simulink model "EMplanner_cs2018a"  (R2018a)
settings: Solver=ode5  StartTime=0.0  StopTime=50  FixedStep=1/1000  RelTol=1e-3
PreLoadFcn:
  | mbxruntime.callbacks.PreLoadFcn(bdroot);
PostLoadFcn:
  | mbxruntime.callbacks.PostLoadFcn(bdroot);
InitFcn:
  | mbxruntime.callbacks.InitFcn(bdroot);
StartFcn:
  | mbxruntime.callbacks.StartFcn(bdroot);
StopFcn:
  | mbxruntime.callbacks.StopFcn(bdroot);
model workspace (MAT data in the model file):
  mbox_table : struct (value not decoded)
  model_closed = 0
  sim_status = 0
values from neighbouring files (symbols this model uses):
  c_factor = 43.75    [emplanner_init.m]
  cf = -175016    [emplanner_init.m]
  cr = -130634    [emplanner_init.m]
  global_path_x = [-2.9245 -1.92511774493 -0.926994634419 0.0698522493473 1.06541712279 2.05969835808 3.05269585569 4.04441007764 5.03484169183 6.02399144113 7.01186009523 7.99844843293 ... (1201 elements, 1201x1)]    [global_path.mat]
  global_path_y = [13.2143 13.2143 13.2143 13.2143 13.2143 13.2143 13.2143 13.2143 13.2143 13.2143 13.2143 13.2143 ... (1201 elements, 1201x1)]    [global_path.mat]
  KD_PID_distance = 0.0    (= 0)    [emplanner_init.m]
  KD_PID_speed = 0    [emplanner_init.m]
  KI_PID_distance = 0.0    (= 0)    [emplanner_init.m]
  KI_PID_speed = 0    [emplanner_init.m]
  KP_PID_distance = 0.5    [emplanner_init.m]
  KP_PID_speed = 1.8    [emplanner_init.m]
  la = 1.265    [emplanner_init.m]
  lb = 2.947-1.265    (= 1.682)    [emplanner_init.m]
  LQR_K1 = k(:,1)'    [emplanner_init.m]
  LQR_K2 = k(:,2)'    [emplanner_init.m]
  LQR_K3 = k(:,3)'    [emplanner_init.m]
  LQR_K4 = k(:,4)'    [emplanner_init.m]
  m = 2020    [emplanner_init.m]
  rack_displacement = [-39.14 , -37.2 , -35.29 , -33.43 , -31.6 , -29.81 , -28.06 , -26.34 , -24.66 ,      -23.01 , -21.38 , -19.79 , -18.23 , -16.69 , -15.18 , -13.7 , -12.23 , -10.8 , -9.38 , -7.98 ,     -6.61 , -5.25 , -3.91 , -2.59 , -1.29 , 0 , 1.27 , 2.54 , 3.78 , 5.02 , 6.24 , 7.46 , 8.66 ,      9.86 , 11.05 , 12.24 , 13.41 , 14.59 , 15.76 , 16.92 , 18.09 , 19.25 , 20.42 , 21.59 , 22.76 ,      23.93 , 25.11 , 26 ...(+26 chars)    [emplanner_init.m]
  right_wheel_ground = [-70 ,-67.2 , -64.4 , -61.6 , -58.8 , -56 , -53.2 , -50.4 , -47.6 , -44.8 , -42 ,      -39.2 , -36.4 , -33.6 , -30.8 , -28 , -25.2 , -22.4 , -19.6 , -16.8 , -14 , -11.2 , -8.4 , -5.6 ,      -2.8 , 0 , 2.8 , 5.6 , 8.4 , 11.2 , 14 , 16.8 , 19.6 , 22.4 , 25.2 , 28 , 30.8 , 33.6 , 36.4 ,      39.2 , 42 , 44.8 , 47.6 , 50.4 , 53.2 , 56 , 58.8 , 61.6 , 64.4 , 67.2 , 70 ]    [emplanner_init.m]
  vx_break_point = zeros(1,5000)    [emplanner_init.m]
undefined symbols (not defined in the file or in its folder): aubr, DiscIntNeverNeededParam, tablebr, vubr, warningInitialVelocity, x0
libraries: simulink x19, simulink_extras x5, PreScanSimulinkLibrary x4, Solver_SF x1
(part 3 of 5)

== system EMplanner_cs2018a/Audi_A8_Sedan_1/control module/control main/chassic steering system ==
  LQR_final_angle : Inport
  Constant : Constant  Value=la
  Constant1 : Constant  Value=lb
  Constant17 : Constant  Value=c_factor
  Divide : Product  Inputs=*/
  Gain3 : Gain  Gain=180/pi
  Gain4 : Gain  Gain=360
  MATLAB Function : MATLAB Function  TreatAsAtomicUnit=on
  Saturation : Saturate  UpperLimit=70  LowerLimit=-70
  Saturation1 : Saturate  UpperLimit=1.2217  LowerLimit=-1.2217
  transfer right wheel angle to rack displancement : Lookup_n-D  NumberOfTableDimensions=1  BreakpointsForDimension1=right_wheel_ground  Table=rack_displacement  InternalRulePriority=Speed  RndMeth=Simplest  InputSameDT=on
  lat_steer_sw[deg] : Outport
  wires:
  transfer right wheel angle to rack displancement/1 -> Divide/1
  Constant17/1 -> Divide/2
  Gain4/1 -> lat_steer_sw[deg]/1
  Divide/1 -> Gain4/1
  Saturation/1 -> transfer right wheel angle to rack displancement/1
  Constant/1 -> MATLAB Function/2(la)
  Gain3/1 -> Saturation/1
  Constant1/1 -> MATLAB Function/3(lb)
  LQR_final_angle/1 -> Saturation1/1
  Saturation1/1 -> MATLAB Function/1(u)
  MATLAB Function/1(right_steer) -> Gain3/1

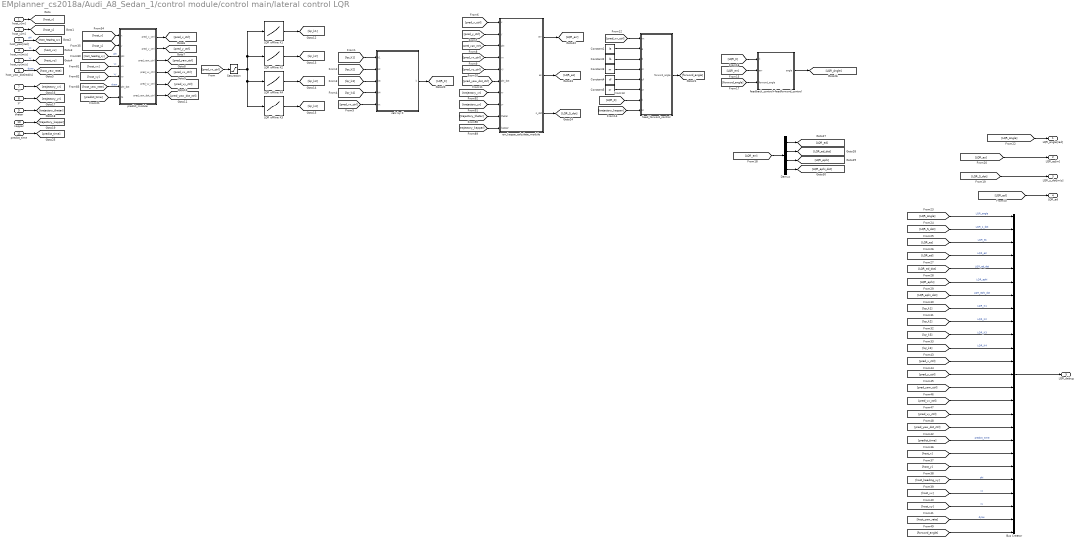
== system EMplanner_cs2018a/Audi_A8_Sedan_1/control module/control main/lateral control LQR ==
  host_x[m] : Inport
  host_y[m] : Inport  Port=2
  host_yaw[rad] : Inport  Port=3
  host_vx[m/s] : Inport  Port=4
  host_vy[m/s] : Inport  Port=5
  host_yaw_dot[rad/s] : Inport  Port=6
  xr : Inport  Port=7
  yr : Inport  Port=8
  thetar : Inport  Port=9
  kappar : Inport  Port=10
  predict_time : Inport  Port=11
  Bus Creator : BusCreator  Inputs=25
  Constant1 : Constant  Value=la
  Constant2 : Constant  Value=lb
  Constant3 : Constant  Value=m
  Constant4 : Constant  Value=cf
  Constant5 : Constant  Value=cr
  Demux : Demux
  LQR offline K1 : Lookup_n-D  NumberOfTableDimensions=1  BreakpointsForDimension1=vx_break_point  Table=LQR_K1  InternalRulePriority=Speed  RndMeth=Simplest  InputSameDT=on
  LQR offline K2 : Lookup_n-D  NumberOfTableDimensions=1  BreakpointsForDimension1=vx_break_point  Table=LQR_K2  InternalRulePriority=Speed  RndMeth=Simplest  InputSameDT=on
  LQR offline K3 : Lookup_n-D  NumberOfTableDimensions=1  BreakpointsForDimension1=vx_break_point  Table=LQR_K3  InternalRulePriority=Speed  RndMeth=Simplest  InputSameDT=on
  LQR offline K4 : Lookup_n-D  NumberOfTableDimensions=1  BreakpointsForDimension1=vx_break_point  Table=LQR_K4  InternalRulePriority=Speed  RndMeth=Simplest  InputSameDT=on
  Saturation : Saturate  UpperLimit=50  LowerLimit=0
  calc lqr K : MATLAB Function  TreatAsAtomicUnit=on
  err_kappa_calculate_module : MATLAB Function  TreatAsAtomicUnit=on
  feed_forword_control : MATLAB Function  TreatAsAtomicUnit=on
  feedback_control+feedforword_control : MATLAB Function  TreatAsAtomicUnit=on
  predict_module : MATLAB Function  TreatAsAtomicUnit=on
  LQR_angle[rad] : Outport  VectorParamsAs1DForOutWhenUnconnected=off
  LQR_es[m] : Outport  Port=2  VectorParamsAs1DForOutWhenUnconnected=off
  LQR_s_dot[m/s] : Outport  Port=3  VectorParamsAs1DForOutWhenUnconnected=off
  LQR_ed : Outport  Port=4  VectorParamsAs1DForOutWhenUnconnected=off
  LQR_debug : Outport  Port=5  VectorParamsAs1DForOutWhenUnconnected=off
  wires:
  [host_vy] -> predict_module/5(vy)  "vy"
  [host_x] -> predict_module/1(x)
  [host_yaw_rate] -> predict_module/6(phi_dot)  "dyaw"
  [host_vx] -> predict_module/4(vx)  "vx"
  [host_y] -> predict_module/2(y)
  [host_heading_xy] -> predict_module/3(phi)  "phi"
  [predict_time] -> predict_module/7(ts)
  host_x[m]/1 -> [host_x]
  host_y[m]/1 -> [host_y]
  host_yaw[rad]/1 -> [host_heading_xy]  "phi"
  host_vx[m/s]/1 -> [host_vx]  "vx"
  host_vy[m/s]/1 -> [host_vy]  "vy"
  host_yaw_dot[rad/s]/1 -> [host_yaw_rate]  "dyaw"
  predict_module/1(pred_x_ctrl) -> [pred_x_ctrl]
  predict_module/2(pred_y_ctrl) -> [pred_y_ctrl]
  predict_module/3(pred_yaw_ctrl) -> [pred_yaw_ctrl]
  predict_module/4(pred_vx_ctrl) -> [pred_vx_ctrl]
  predict_module/5(pred_vy_ctrl) -> [pred_vy_ctrl]
  predict_module/6(pred_yaw_dot_ctrl) -> [pred_yaw_dot_ctrl]
  [pred_vx_ctrl] -> Saturation/1
  LQR offline K1/1 -> [lqr_k1]
  LQR offline K2/1 -> [lqr_k2]
  LQR offline K4/1 -> [lqr_k3]
  LQR offline K3/1 -> [lqr_k4]
  [pred_vx_ctrl] -> calc lqr K/5(vx)
  [lqr_k4] -> calc lqr K/4(k4)
  [lqr_k3] -> calc lqr K/3(k3)
  [lqr_k2] -> calc lqr K/2(k2)
  [lqr_k1] -> calc lqr K/1(k1)
  [pred_x_ctrl] -> err_kappa_calculate_module/1(x)
  [pred_y_ctrl] -> err_kappa_calculate_module/2(y)
  [pred_yaw_ctrl] -> err_kappa_calculate_module/3(phi)
  [pred_vx_ctrl] -> err_kappa_calculate_module/4(vx)
  [pred_vy_ctrl] -> err_kappa_calculate_module/5(vy)
  [pred_yaw_dot_ctrl] -> err_kappa_calculate_module/6(phi_dot)
  xr/1 -> [trajectory_xr]
  yr/1 -> [trajectory_yr]
  thetar/1 -> [trajectory_thetar]
  kappar/1 -> [trajectory_kappar]
  [trajectory_xr] -> err_kappa_calculate_module/7(xr)
  [trajectory_yr] -> err_kappa_calculate_module/8(yr)
  [trajectory_kappar] -> err_kappa_calculate_module/10(kappar)
  [trajectory_thetar] -> err_kappa_calculate_module/9(thetar)
  [pred_vx_ctrl] -> feed_forword_control/1(vx)
  Constant1/1 -> feed_forword_control/2(a)
  Constant2/1 -> feed_forword_control/3(b)
  Constant3/1 -> feed_forword_control/4(m)
  Constant4/1 -> feed_forword_control/5(cf)
  Constant5/1 -> feed_forword_control/6(cr)
  calc lqr K/1(k) -> [LQR_K]
  [LQR_K] -> feed_forword_control/7(k)
  [trajectory_kappar] -> feed_forword_control/8(kr)
  feed_forword_control/1(forword_angle) -> [forword_angle]
  err_kappa_calculate_module/1(err) -> [LQR_err]
  [LQR_err] -> feedback_control+feedforword_control/2(err)
  [LQR_K] -> feedback_control+feedforword_control/1(k)
  [forword_angle] -> feedback_control+feedforword_control/3(forword_angle)
  [LQR_err] -> Demux/1
  err_kappa_calculate_module/2(es) -> [LQR_es]
  err_kappa_calculate_module/3(s_dot) -> [LQR_S_dot]
  [LQR_S_dot] -> LQR_s_dot[m/s]/1
  [LQR_es] -> LQR_es[m]/1
  Saturation/1 -> LQR offline K3/1, LQR offline K4/1, LQR offline K2/1, LQR offline K1/1
  predict_time/1 -> [predict_time]
  Bus Creator/1 -> LQR_debug/1
  feedback_control+feedforword_control/1(angle) -> [LQR_Angle]
  [LQR_Angle] -> LQR_angle[rad]/1
  [LQR_Angle] -> Bus Creator/1  "LQR_angle"
  [LQR_S_dot] -> Bus Creator/2  "LQR_s_dot"
  [LQR_es] -> Bus Creator/3  "LQR_es"
  Demux/1 -> [LQR_ed]
  Demux/2 -> [LQR_ed_dot]
  Demux/3 -> [LQR_ephi]
  Demux/4 -> [LQR_ephi_dot]
  [LQR_ed] -> Bus Creator/4  "LQR_ed"
  [LQR_ed_dot] -> Bus Creator/5  "LQR_ed_dot"
  [LQR_ephi] -> Bus Creator/6  "LQR_ephi"
  [LQR_ephi_dot] -> Bus Creator/7  "LQR_ephi_dot"
  [lqr_k1] -> Bus Creator/8  "LQR_K1"
  [lqr_k2] -> Bus Creator/9  "LQR_K2"
  [lqr_k3] -> Bus Creator/10  "LQR_K3"
  [lqr_k4] -> Bus Creator/11  "LQR_K4"
  [pred_x_ctrl] -> Bus Creator/12
  [pred_y_ctrl] -> Bus Creator/13
  [pred_yaw_ctrl] -> Bus Creator/14
  [pred_vx_ctrl] -> Bus Creator/15
  [pred_vy_ctrl] -> Bus Creator/16
  [pred_yaw_dot_ctrl] -> Bus Creator/17
  [predict_time] -> Bus Creator/18  "predict_time"
  [host_x] -> Bus Creator/19
  [host_y] -> Bus Creator/20
  [host_heading_xy] -> Bus Creator/21  "phi"
  [host_vx] -> Bus Creator/22  "vx"
  [host_vy] -> Bus Creator/23  "vy"
  [host_yaw_rate] -> Bus Creator/24  "dyaw"
  [forword_angle] -> Bus Creator/25
  [LQR_ed] -> LQR_ed/1

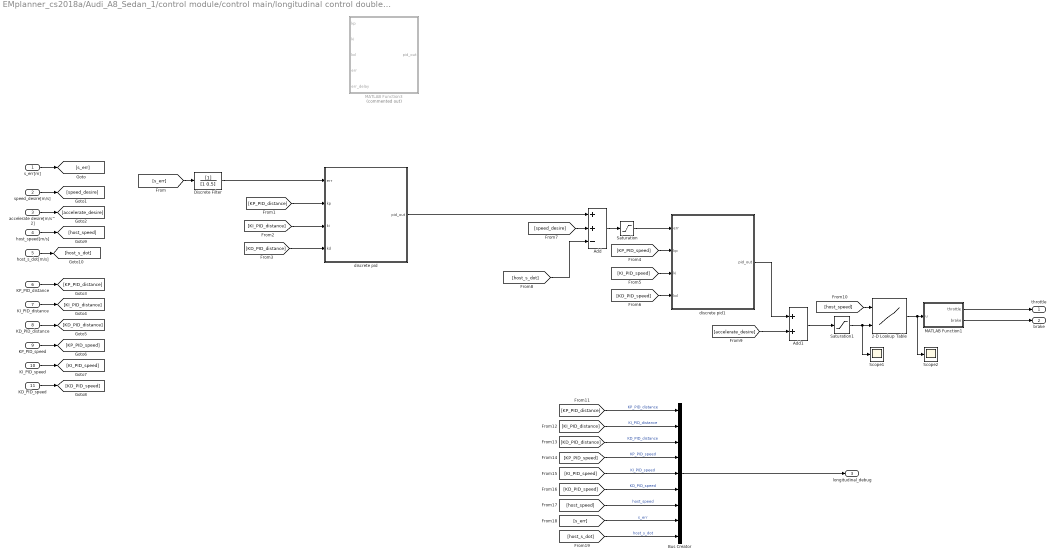
== system EMplanner_cs2018a/Audi_A8_Sedan_1/control module/control main/longitudinal control double PID ==
  s_err[m] : Inport
  speed_desire[m/s] : Inport  Port=2
  accelerate desire[m/s^2] : Inport  Port=3
  host_speed[m/s] : Inport  Port=4
  host_s_dot[m/s] : Inport  Port=5
  KP_PID_distance : Inport  Port=6
  KI_PID_distance : Inport  Port=7
  KD_PID_distance : Inport  Port=8
  KP_PID_speed : Inport  Port=9
  KI_PID_speed : Inport  Port=10
  KD_PID_speed : Inport  Port=11
  2-D Lookup Table : Lookup_n-D  BreakpointsForDimension1=vubr  BreakpointsForDimension2=aubr  Table=tablebr  InternalRulePriority=Speed  RndMeth=Simplest  InputSameDT=on
  Add : Sum  Inputs=++-
  Add1 : Sum
  Bus Creator : BusCreator  Inputs=9
  Discrete Filter : DiscreteFilter
  MATLAB Function1 : MATLAB Function  TreatAsAtomicUnit=on
  MATLAB Function3 : MATLAB Function  Commented=on  TreatAsAtomicUnit=on
  Saturation : Saturate  UpperLimit=45  LowerLimit=-45
  Saturation1 : Saturate  UpperLimit=5  LowerLimit=-8
  Scope1 : Scope
  Scope2 : Scope
  discrete pid : Subsystem
  discrete pid1 : Subsystem
  throttle : Outport
  brake : Outport  Port=2
  longitudinal_debug : Outport  Port=3
  wires:
  2-D Lookup Table/1 -> Scope2/1, MATLAB Function1/1(u)
  s_err[m]/1 -> [s_err]
  speed_desire[m/s]/1 -> [speed_desire]
  accelerate desire[m/s^2]/1 -> [accelerate_desire]
  KP_PID_distance/1 -> [KP_PID_distance]
  KI_PID_distance/1 -> [KI_PID_distance]
  KD_PID_distance/1 -> [KD_PID_distance]
  KP_PID_speed/1 -> [KP_PID_speed]
  KI_PID_speed/1 -> [KI_PID_speed]
  KD_PID_speed/1 -> [KD_PID_speed]
  [s_err] -> Discrete Filter/1
  host_speed[m/s]/1 -> [host_speed]
  [speed_desire] -> Add/2
  Add/1 -> Saturation/1
  Saturation/1 -> discrete pid1/1(err)
  discrete pid1/1(pid_out) -> Add1/1
  [accelerate_desire] -> Add1/2
  Add1/1 -> Saturation1/1
  Saturation1/1 -> Scope1/1, 2-D Lookup Table/2
  host_s_dot[m/s]/1 -> [host_s_dot]
  [host_s_dot] -> Add/3
  [host_speed] -> 2-D Lookup Table/1
  MATLAB Function1/1(throttle) -> throttle/1
  MATLAB Function1/2(brake) -> brake/1
  [KP_PID_distance] -> Bus Creator/1  "KP_PID_distance"
  [KI_PID_distance] -> Bus Creator/2  "KI_PID_distance"
  [KD_PID_distance] -> Bus Creator/3  "KD_PID_distance"
  [KP_PID_speed] -> Bus Creator/4  "KP_PID_speed"
  [KI_PID_speed] -> Bus Creator/5  "KI_PID_speed"
  [KD_PID_speed] -> Bus Creator/6  "KD_PID_speed"
  [host_speed] -> Bus Creator/7  "host_speed"
  [s_err] -> Bus Creator/8  "s_err"
  [host_s_dot] -> Bus Creator/9  "host_s_dot"
  Bus Creator/1 -> longitudinal_debug/1
  discrete pid/1(pid_out) -> Add/1
  Discrete Filter/1 -> discrete pid/1(err)
  [KP_PID_distance] -> discrete pid/2(kp)
  [KI_PID_distance] -> discrete pid/3(ki)
  [KD_PID_distance] -> discrete pid/4(kd)
  [KP_PID_speed] -> discrete pid1/2(kp)
  [KI_PID_speed] -> discrete pid1/3(ki)
  [KD_PID_speed] -> discrete pid1/4(kd)

== system EMplanner_cs2018a/Audi_A8_Sedan_1/control module/control main/understeer compensate ==
  LQR_angle : Inport
  lateral err : Inport  Port=2
  Add : Sum  Inputs=+-
  Gain : Gain  Gain=0.01
  Manual Switch : ManualSwitch
  LQR_final_angle : Outport
  wires:
  lateral err/1 -> Gain/1
  Add/1 -> Manual Switch/2
  Manual Switch/1 -> LQR_final_angle/1
  LQR_angle/1 -> Add/1, Manual Switch/1
  Gain/1 -> Add/2

== system EMplanner_cs2018a/Audi_A8_Sedan_2/Dynamics_Simple/Chassis/Bicycle_model_[XYZ] ==
  DeltaWheel_[rad] : Inport
  zFront_[m]_dzFront_[ms-1] : Inport  Port=2  PortDimensions=2
  zRear_[m]_dzRear_[ms-1] : Inport  Port=3  PortDimensions=2
  BrakePressure_[bar] : Inport  Port=4
  DriveTorque_[Nm] : Inport  Port=5
  v0_[ms-1] : Inport  Port=6
  |vx|_[ms-1] : Inport  Port=7
  Fy_rear_[N] : Inport  Port=8
  Fy_front_[N] : Inport  Port=9
  Demux : Demux  Outputs=2
  Demux1 : Demux  Outputs=2
  Fyi --> Fy / Mz : Subsystem
  X_Motion : Subsystem
  Y & Yaw_Motion : Subsystem
  "Z, Pitch_Motion & Roll_Motion" : Subsystem
  |vx|_[ms-1]1 : Outport
  vy_[ms-1] : Outport  Port=2
  vz_[ms-1] : Outport  Port=3
  RollAngle_[rad] : Outport  Port=4
  RollRate_[rads-1] : Outport  Port=5
  YawAngle_[rads-1] : Outport  Port=6
  Vx_[ms-1] : Outport  Port=7
  PitchAngle_[rad] : Outport  Port=8
  YawAngle_[rad] : Outport  Port=9
  ax_[ms-2] : Outport  Port=10
  ay_[ms-2] : Outport  Port=11
  wires:
  Fyi --> Fy / Mz/1(Fy_[N]) -> Y & Yaw_Motion/2(Fy_[N])  "Fy_[N]"
  Fyi --> Fy / Mz/2(Mz_[Nm]) -> Y & Yaw_Motion/3(Mz_[Nm])  "Mz_[Nm]"
  Y & Yaw_Motion/1(|vx|_[ms-1]1) -> |vx|_[ms-1]1/1  "|vx|_[ms-1]"
  Y & Yaw_Motion/2(vy_[ms-1]) -> vy_[ms-1]/1  "vy_[ms-1]"
  Y & Yaw_Motion/5(YawAngle_[rad]) -> YawAngle_[rad]/1  "YawAngle_[rad]"
  v0_[ms-1]/1 -> X_Motion/3(v0_[ms-1])  "v0_[ms-1]"
  BrakePressure_[bar]/1 -> X_Motion/2(BrakePressure_[bar])  "BrakePressure_[bar]"
  DriveTorque_[Nm]/1 -> X_Motion/1(DriveTorque_[Nm])  "DriveTorque_[Nm]"
  X_Motion/2(ax_[ms-2]) -> ax_[ms-2]/1, [ax]  "ax_[ms-2]"
  X_Motion/1(vx_[ms-1]) -> Vx_[ms-1]/1, [vx]  "vx_[ms-1]"
  [ax] -> "Z, Pitch_Motion & Roll_Motion"/3(ax)
  Demux/1 -> "Z, Pitch_Motion & Roll_Motion"/5(zFront_[m])
  Demux/2 -> "Z, Pitch_Motion & Roll_Motion"/6(dzFront_[ms-1])
  Demux1/1 -> "Z, Pitch_Motion & Roll_Motion"/7(zRear_[m])
  Demux1/2 -> "Z, Pitch_Motion & Roll_Motion"/8(dzRear_[ms-1])
  zRear_[m]_dzRear_[ms-1]/1 -> Demux1/1
  zFront_[m]_dzFront_[ms-1]/1 -> Demux/1
  "Z, Pitch_Motion & Roll_Motion"/2(vz_[ms-1]) -> vz_[ms-1]/1  "vz_[ms-1]"
  DeltaWheel_[rad]/1 -> Fyi --> Fy / Mz/1(DeltaWheel_[rad])
  Fy_front_[N]/1 -> Fyi --> Fy / Mz/2(Fy_f_[N])
  Fy_rear_[N]/1 -> Fyi --> Fy / Mz/3(Fy_r_[N])
  |vx|_[ms-1]/1 -> Y & Yaw_Motion/1(|vx|_[ms-1])
  Y & Yaw_Motion/3(ay_[ms-2]) -> [ay], ay_[ms-2]/1  "ay_[ms-2]"
  [ay] -> "Z, Pitch_Motion & Roll_Motion"/4(ay)
  "Z, Pitch_Motion & Roll_Motion"/3(RollAngle_[rad]) -> RollAngle_[rad]/1  "RollAngle_[rad]"
  "Z, Pitch_Motion & Roll_Motion"/4(RollRate_[rads-1]) -> RollRate_[rads-1]/1  "RollRate_[rads-1]"
  [dYaw] -> "Z, Pitch_Motion & Roll_Motion"/2(dYaw)
  [vx] -> "Z, Pitch_Motion & Roll_Motion"/1(vx)
  Y & Yaw_Motion/4(dYawAngle_[rads-1]) -> YawAngle_[rads-1]/1, [dYaw]  "dYawAngle_[rads-1]"
  "Z, Pitch_Motion & Roll_Motion"/1(pitchAngle_[rad]) -> PitchAngle_[rad]/1  "PitchAngle_[rad]"

== system EMplanner_cs2018a/Audi_A8_Sedan_2/Dynamics_Simple/Chassis/FrontTyre ==
  note: alpha limiter
      | [-1 ... 1]
  note: relax_on
      | ON: 1
      | OFF: 0
  note: MOTORCYCLE ONLY
  note: VEHICLE + MOTORCYCLE
  DeltaWheel_[rad] : Inport
  |vx|_[ms-1] : Inport  Port=2
  vy_[ms-1] : Inport  Port=3
  dYawAngle_[rads-1] : Inport  Port=4
  RollAngle_[rad] : Inport  Port=5
  AlphaFront : Subsystem
  Compare To Zero : simulink/Logic and Bit Operations/Compare To Zero  relop===  OutDataTypeStr=boolean  ZeroCross=off
  Configurable Subsystem : Subsystem  BlockChoice=Integrator  mask{ComputationMode=ComputationMode}
      mask prompts: ComputationMode "Computation mode:"
      mask init:
      | SetComputationMode(gcb,ComputationMode);
      settings: AttributesFormatString=%<BlockChoice>  OpenFcn=BringToFront(gcb);  MemberBlocks=Discrete-Time Integrator,Integrator
      settings: TemplateBlock=|
      | PreScanSimulinkLibrary/Configurable Subsystems/integral with reset and limits
      | for slip angle/Configurable
      | Subsystem
  Configurable Subsystem1 : Subsystem  BlockChoice=Integrator  mask{ComputationMode=ComputationMode}
      mask prompts: ComputationMode "Computation mode:"
      mask init:
      | SetComputationMode(gcb,ComputationMode);
      settings: AttributesFormatString=%<BlockChoice>  OpenFcn=BringToFront(gcb);  MemberBlocks=Discrete-Time Integrator,Integrator
      settings: TemplateBlock=|
      | PreScanSimulinkLibrary/Configurable Subsystems/integral with reset/Configurable
      | Subsystem
  Constant : Constant  Value=p.relax_on
  Constant1 : Constant  Value=p.relax_on
  Constant2 : Constant  Value=p.VehMCSwitch
  Data Type Conversion : DataTypeConversion  OutDataTypeStr=double
  If MC : simulink/Logic and Bit Operations/Compare To Constant  relop===  const=2  OutDataTypeStr=uint8  ZeroCross=off
  K_gamma_front : Gain  Gain=p.Kgfront
  Linl : Fcn  Expr=(u(4) - u(5))/p.sigma_front*u(1)
  Linl1 : Fcn  Expr=(u(4) - u(5))/p.sigma_front*u(1)
  Mux1 : Mux  Inputs=3
  Mux2 : Mux  Inputs={3,1,1}
  Mux3 : Mux  Inputs={3,1,1}
  Prevent_instability_at_low_Vx : Subsystem
  Product : Product  RndMeth=Zero
  Sum : Sum  Inputs=|++  InputSameDT=on  SaturateOnIntegerOverflow=on  OutDataTypeStr=Inherit: Same as first input
  Sum1 : Sum  Inputs=|++
  Switch : Switch  Threshold=0.5  SaturateOnIntegerOverflow=on  InputSameDT=on
  Switch1 : Switch  Threshold=0.5  SaturateOnIntegerOverflow=on  InputSameDT=on
  alg.loop : Memory
  due to sign convention : Gain  Gain=-1  SaturateOnIntegerOverflow=on  OutDataTypeStr=Inherit: Same as input  ParamDataTypeStr=Inherit: Same as input
  front_tyre : Gain  Gain=p.Kfront
  FyFront_[N] : Outport
  wires:
  Prevent_instability_at_low_Vx/1(alpha [rad]) -> Mux2/2, Switch/3
  Sum/1 -> Prevent_instability_at_low_Vx/1(alpha[rad])  "AlphaStatFront_[rad]"
  Switch/1 -> front_tyre/1  "AlphaFront_[rad]"
  Constant/1 -> Switch/2
  Sum1/1 -> FyFront_[N]/1  "FyFront_[N]"
  Mux2/1 -> Linl/1
  Linl/1 -> Configurable Subsystem/1(In1)
  Configurable Subsystem/1(Out1) -> Mux2/3, Switch/1  "AlphaRelaxFront_[rad]"
  AlphaFront/1(Alpha) -> Sum/1
  Mux1/1 -> Prevent_instability_at_low_Vx/2(In), AlphaFront/1(In), Mux2/1, Mux3/1
  |vx|_[ms-1]/1 -> Mux1/1, Compare To Zero/1
  vy_[ms-1]/1 -> Mux1/2
  dYawAngle_[rads-1]/1 -> Mux1/3
  alg.loop/1 -> Switch1/3
  Configurable Subsystem1/1(Out1) -> Mux3/3, Switch1/1  "GammaRelaxFront_[rad]"
  Linl1/1 -> Configurable Subsystem1/1(In1)
  Mux3/1 -> Linl1/1
  Constant1/1 -> Switch1/2
  due to sign convention/1 -> alg.loop/1, Mux3/2  "GammaStatFront_[rad]"
  RollAngle_[rad]/1 -> due to sign convention/1
  front_tyre/1 -> Sum1/1
  Constant2/1 -> If MC/1
  If MC/1 -> Data Type Conversion/1
  K_gamma_front/1 -> Product/1
  Product/1 -> Sum1/2
  Data Type Conversion/1 -> Product/2
  Compare To Zero/1 -> [reset]
  [reset] -> Configurable Subsystem/2(In2)
  [reset] -> Configurable Subsystem1/2(In2)
  DeltaWheel_[rad]/1 -> Sum/2  "DeltaWheel_[rad]"
  Switch1/1 -> K_gamma_front/1  "GammaFront_[rad]"

== system EMplanner_cs2018a/Audi_A8_Sedan_2/Dynamics_Simple/Chassis/MuxDynState ==
  note: The position inputs are computed by the
      | integrated velocity.
  note: mode: Dynamics
      | VelVEHICLE
      | wrt VEH
  note: AnglesVEHICLE
      | wrtGLOB
  vx [ms-1] : Inport
  vy [ms-1] : Inport  Port=2
  vz [ms-1] : Inport  Port=3
  R [rad] : Inport  Port=4
  P [rad] : Inport  Port=5
  Y [rad] : Inport  Port=6
  Configurable Subsystem1 : Subsystem  BlockChoice=Integrator  mask{ComputationMode=ComputationMode}
      mask prompts: ComputationMode "Computation mode:"
      mask init:
      | SetComputationMode(gcb,ComputationMode);
      settings: AttributesFormatString=%<BlockChoice>  OpenFcn=BringToFront(gcb);  MemberBlocks=Discrete-Time Integrator,Integrator
      settings: TemplateBlock=|
      | PreScanSimulinkLibrary/Configurable Subsystems/integral/Configurable
      | Subsystem1
  Ground : Ground
  Ground1 : Ground
  Mux : Mux  Inputs=[3 3 3]
  Mux1 : Mux  Inputs=3
  Mux2 : Mux  Inputs=3
  Transformation_BODY2GLOBAL : Subsystem
  mux3 : Mux  Inputs=3
  State : Outport
  wires:
  Ground1/1 -> mux3/2  "pitch"
  Y [rad]/1 -> Mux2/3, mux3/3  "yaw"
  P [rad]/1 -> Mux2/2
  R [rad]/1 -> Mux2/1
  vz [ms-1]/1 -> Mux1/3
  vy [ms-1]/1 -> Mux1/2
  vx [ms-1]/1 -> Mux1/1
  Mux2/1 -> Mux/3
  Transformation_BODY2GLOBAL/1(Vvector_GLOBAL_[m/s]) -> Configurable Subsystem1/1(In1), Mux/2  "VelVEH wrt  GLOB"
  mux3/1 -> Transformation_BODY2GLOBAL/2(angles_BODYwrtGLOB_[rad])
  Ground/1 -> mux3/1  "roll"
  Mux/1 -> State/1
  Mux1/1 -> Transformation_BODY2GLOBAL/1(Vvector_BODY_[m/s])
  Configurable Subsystem1/1(Out1) -> Mux/1  "PosVEH wrt  GLOB"

== system EMplanner_cs2018a/Audi_A8_Sedan_2/Dynamics_Simple/Chassis/Power Assisted Steering ==
  note: MOTORCYCLE
  note: VEHICLE
  note: Reverse steering direction for negative velocities
  Vx_[ms-1] : Inport
  Delta_in_[deg] : Inport  Port=2
  Constant : Constant
  Constant1 : Constant  Value=p.VehMCSwitch
  Lookup Table : Lookup  InputValues=[0 35 45 100]  Table=[1 1 0.2 0.2]
  Multiport Switch : MultiPortSwitch  Inputs=2
  Product : Product  Inputs=3  RndMeth=Zero
  Sign : Signum
  Delta_out_[deg] : Outport
  wires:
  Vx_[ms-1]/1 -> Lookup Table/1, Sign/1
  Delta_in_[deg]/1 -> Product/3
  Constant1/1 -> Multiport Switch/1
  Constant/1 -> Multiport Switch/3
  Lookup Table/1 -> Multiport Switch/2
  Multiport Switch/1 -> Product/2
  Product/1 -> Delta_out_[deg]/1
  Sign/1 -> Product/1

== system EMplanner_cs2018a/Audi_A8_Sedan_2/Dynamics_Simple/Chassis/RearTyre ==
  note: alpha limiter
      | [-1 ... 1]
  note: relax_on
      | ON: 1
      | OFF: 0
  note: MOTORCYCLE ONLY
  note: VEHICLE + MOTORCYCLE
  |vx|_[ms-1] : Inport
  vy_[ms-1] : Inport  Port=2
  dpsi_[rads-1] : Inport  Port=3
  RollAngle_[rad] : Inport  Port=4
  AlphaRear : Subsystem
  Compare To Zero : simulink/Logic and Bit Operations/Compare To Zero  relop===  OutDataTypeStr=boolean  ZeroCross=off
  Configurable Subsystem : Subsystem  BlockChoice=Integrator  mask{ComputationMode=ComputationMode}
      mask prompts: ComputationMode "Computation mode:"
      mask init:
      | SetComputationMode(gcb,ComputationMode);
      settings: AttributesFormatString=%<BlockChoice>  OpenFcn=BringToFront(gcb);  MemberBlocks=Discrete-Time Integrator,Integrator
      settings: TemplateBlock=|
      | PreScanSimulinkLibrary/Configurable Subsystems/integral with reset/Configurable
      | Subsystem
  Configurable Subsystem1 : Subsystem  BlockChoice=Integrator  mask{ComputationMode=ComputationMode}
      mask prompts: ComputationMode "Computation mode:"
      mask init:
      | SetComputationMode(gcb,ComputationMode);
      settings: AttributesFormatString=%<BlockChoice>  OpenFcn=BringToFront(gcb);  MemberBlocks=Discrete-Time Integrator,Integrator
      settings: TemplateBlock=|
      | PreScanSimulinkLibrary/Configurable Subsystems/integral with reset and limits
      | for slip angle/Configurable
      | Subsystem
  Constant1 : Constant  Value=p.relax_on
  Constant2 : Constant  Value=p.relax_on
  Constant3 : Constant  Value=p.VehMCSwitch
  Data Type Conversion : DataTypeConversion  OutDataTypeStr=double
  If MC : simulink/Logic and Bit Operations/Compare To Constant  relop===  const=2  OutDataTypeStr=uint8  ZeroCross=off
  K_gamma_rear : Gain  Gain=p.Kgrear
  Linl : Fcn  Expr=(u(4) - u(5))/p.sigma_rear*u(1)
  Linl1 : Fcn  Expr=(u(4) - u(5))/p.sigma_rear*u(1)
  Mux1 : Mux  Inputs=3
  Mux2 : Mux  Inputs={3,1,1}
  Mux3 : Mux  Inputs={3,1,1}
  Prevent_instability_at_low_Vx : PreScanSimulinkLibrary/Simple_Vehicle_Dynamics/Chassis/FrontTyre/Prevent_instability_at_low_Vx  SystemSampleTime=-1  Latency=0  AutoFrameSizeCalculation=off
  Product : Product  RndMeth=Zero
  Sum1 : Sum  Inputs=|++
  Switch1 : Switch  Threshold=0.5  SaturateOnIntegerOverflow=on  InputSameDT=on
  Switch2 : Switch  Threshold=0.5  SaturateOnIntegerOverflow=on  InputSameDT=on
  alg.loop : Memory
  due to sign convention : Gain  Gain=-1  SaturateOnIntegerOverflow=on  OutDataTypeStr=Inherit: Same as input  ParamDataTypeStr=Inherit: Same as input
  rear_tyre : Gain  Gain=p.Krear
  FyRear_[N] : Outport
  wires:
  Prevent_instability_at_low_Vx/1 -> Switch1/3, Mux2/2
  AlphaRear/1(Alpha) -> Prevent_instability_at_low_Vx/1  "AlphaStatRear_[rad]"
  Switch1/1 -> rear_tyre/1  "AlphaRear_[rad]"
  Constant1/1 -> Switch1/2
  Sum1/1 -> FyRear_[N]/1  "FyRear_[N]"
  Mux2/1 -> Linl/1
  Linl/1 -> Configurable Subsystem1/1(In1)
  Configurable Subsystem1/1(Out1) -> Mux2/3, Switch1/1  "AlphaRelaxRear_[rad]"
  Mux1/1 -> Prevent_instability_at_low_Vx/2, AlphaRear/1(In), Mux2/1, Mux3/1
  |vx|_[ms-1]/1 -> Mux1/1, Compare To Zero/1
  vy_[ms-1]/1 -> Mux1/2
  dpsi_[rads-1]/1 -> Mux1/3
  alg.loop/1 -> Switch2/3
  Configurable Subsystem/1(Out1) -> Mux3/3, Switch2/1  "GammaRelaxRear_[rad]"
  Linl1/1 -> Configurable Subsystem/1(In1)
  Mux3/1 -> Linl1/1
  Constant2/1 -> Switch2/2
  due to sign convention/1 -> alg.loop/1, Mux3/2  "GammaStatRear_[rad]"
  RollAngle_[rad]/1 -> due to sign convention/1
  Constant3/1 -> If MC/1
  If MC/1 -> Data Type Conversion/1
  Product/1 -> Sum1/2
  Data Type Conversion/1 -> Product/2
  K_gamma_rear/1 -> Product/1
  rear_tyre/1 -> Sum1/1
  Compare To Zero/1 -> [reset]
  [reset] -> Configurable Subsystem1/2(In2)
  [reset] -> Configurable Subsystem/2(In2)
  Switch2/1 -> K_gamma_rear/1  "GammaFront_[rad]"

== system EMplanner_cs2018a/Audi_A8_Sedan_2/Dynamics_Simple/Engine/Configurable Subsystem ==
  In1 : Inport
  Rate Limiter : TransferFcn  Denominator=[0.1 1]
  Out1 : Outport
  wires:
  In1/1 -> Rate Limiter/1
  Rate Limiter/1 -> Out1/1

== system EMplanner_cs2018a/Audi_A8_Sedan_2/Dynamics_Simple/Engine/Configurable Subsystem1 ==
  In1 : Inport
  Integrator : Integrator  InitialCondition=p.rot_ini  LimitOutput=on  UpperSaturationLimit=p.rot_upp  LowerSaturationLimit=p.rot_low
  Out1 : Outport
  wires:
  In1/1 -> Integrator/1
  Integrator/1 -> Out1/1

== system EMplanner_cs2018a/Audi_A8_Sedan_2/Dynamics_Simple/Gear: Auto Manual/If Action Subsystem ==
  In1 : Inport
  Action Port : ActionPort  PropagateVarSize=During execution
  Out1 : Outport
  wires:
  In1/1 -> Out1/1

== system EMplanner_cs2018a/Audi_A8_Sedan_2/Dynamics_Simple/Gear: Auto Manual/If Action Subsystem1 ==
  In1 : Inport
  Action Port : ActionPort  PropagateVarSize=During execution
  Out1 : Outport
  wires:
  In1/1 -> Out1/1

== system EMplanner_cs2018a/Audi_A8_Sedan_2/Dynamics_Simple/ShiftLogic/Detect Increase ==
  GearNr_[-] : Inport
  In2 : Inport  Port=2
  Constant : Constant
  Data Type Conversion : DataTypeConversion  OutDataTypeStr=double
  Data Type Conversion1 : DataTypeConversion  OutDataTypeStr=double
  Detect Increase : simulink/Logic and Bit Operations/Detect Increase  vinit=1  OutDataTypeStr=uint8
  If : If  NumInputs=2  IfExpression="u1==1 &  u2==1"
  If V0 higher of the from 2->3 shifting velocity : Subsystem  TreatAsAtomicUnit=on
  Merge : Merge
  Other : Subsystem  TreatAsAtomicUnit=on
  Out1 : Outport
  wires:
  If/2 -> Other/Action
  If V0 higher of the from 2->3 shifting velocity/1(Out1) -> Merge/1
  Other/1(Out1) -> Merge/2
  Detect Increase/1 -> Data Type Conversion/1
  Merge/1 -> Out1/1
  If/1 -> If V0 higher of the from 2->3 shifting velocity/Action
  Data Type Conversion1/1 -> If/2
  Data Type Conversion/1 -> If/1
  Constant/1 -> If V0 higher of the from 2->3 shifting velocity/1(In1)
  GearNr_[-]/1 -> Detect Increase/1
  In2/1 -> Data Type Conversion1/1, Other/1(In1)

== system EMplanner_cs2018a/Audi_A8_Sedan_2/Dynamics_Simple/ShiftLogic/If Action Neutral ==
  In1 : Inport
  Action Port : ActionPort  InitializeStates=reset  PropagateVarSize=During execution
  Out1 : Outport
  wires:
  In1/1 -> Out1/1

== system EMplanner_cs2018a/Audi_A8_Sedan_2/Dynamics_Simple/ShiftLogic/If Action Normal ==
  In1 : Inport
  Action Port : ActionPort  InitializeStates=reset  PropagateVarSize=During execution
  Out1 : Outport
  wires:
  In1/1 -> Out1/1

== system EMplanner_cs2018a/Audi_A8_Sedan_2/Dynamics_Simple/ShiftLogic/If Action Reverse ==
  In1 : Inport
  Action Port : ActionPort  InitializeStates=reset  PropagateVarSize=During execution
  Out1 : Outport
  wires:
  In1/1 -> Out1/1

== system EMplanner_cs2018a/Audi_A8_Sedan_2/Dynamics_Simple/Transmission/Torque_Converter ==
  note: <= 0
  note: > 0
  note: To compensate for no hydraulic connection when in neutral gear
  nEngine_[rpm] : Inport
  nTransmission_[rpm] : Inport  Port=2
  Gear nr : Inport  Port=3
  Compare To Constant : simulink/Logic and Bit Operations/Compare To Constant  relop=<=  const=1  OutDataTypeStr=uint8  ZeroCross=off
  Compare To Zero : simulink/Logic and Bit Operations/Compare To Zero  relop=~=  OutDataTypeStr=uint8  ZeroCross=off
  Constant : Constant  Value=1/50
  Constant1 : Constant
  Constant2 : Constant
  Drag : Gain  Gain=-1
  FactorK : Lookup  InputValues=p.speedratio  Table=p.Kfactor*p.Kcorr  SaturateOnIntegerOverflow=on
  Impeller : Fcn  Expr=u^2
  Product : Product  RndMeth=Zero
  Product1 : Product  RndMeth=Zero
  Quotient : Product  Inputs=*/  InputSameDT=on  SaturateOnIntegerOverflow=on  OutDataTypeStr=Inherit: Same as first input
  SpeedRatio : Product  Inputs=*/  InputSameDT=on  SaturateOnIntegerOverflow=on  OutDataTypeStr=Inherit: Same as first input
  Sum : Sum  Inputs=|+-
  Switch : Switch  Criteria=u2 ~= 0  Threshold=0.5
  Switch1 : Switch  Criteria=u2 ~= 0
  TorqueRatio : Lookup  InputValues=[p.speedratio 1]  Table=[p.Torqueratio 0]  SaturateOnIntegerOverflow=on
  Turbine : Product  InputSameDT=on  SaturateOnIntegerOverflow=on  OutDataTypeStr=Inherit: Same as first input
  rpm2rads-1 : Gain  Gain=2*pi/60
  ImpellerTorque_[Nm] : Outport  InitialOutput=0
  TurbineTorque_[Nm] : Outport  Port=2  InitialOutput=0
  wires:
  rpm2rads-1/1 -> Quotient/1
  Turbine/1 -> Switch1/1
  TorqueRatio/1 -> Turbine/2
  Compare To Constant/1 -> Switch1/2
  Constant2/1 -> Sum/2
  Sum/1 -> Drag/1
  Drag/1 -> Switch1/3
  Product1/1 -> TurbineTorque_[Nm]/1
  Switch1/1 -> Product1/2
  Compare To Zero/1 -> Switch/2
  Gear nr/1 -> Compare To Zero/1
  Constant1/1 -> Switch/1
  Constant/1 -> Switch/3
  Switch/1 -> Product1/1, Product/1
  Product/1 -> ImpellerTorque_[Nm]/1
  Quotient/1 -> Impeller/1
  FactorK/1 -> Quotient/2
  SpeedRatio/1 -> FactorK/1, Sum/1, Compare To Constant/1, TorqueRatio/1
  Impeller/1 -> Turbine/1, Product/2
  nEngine_[rpm]/1 -> SpeedRatio/2, rpm2rads-1/1
  nTransmission_[rpm]/1 -> SpeedRatio/1

== system EMplanner_cs2018a/Audi_A8_Sedan_2/Dynamics_Simple/Transmission/Transmission_Ratio ==
  tTransmissionIn_[Nm] : Inport
  GearNr_[-] : Inport  Port=2
  nTransmissionOut_[rpm] : Inport  Port=3
  Ensure positive TransmissionRPM : Abs
  If : If  IfExpression=u1 == 0  ElseIfExpressions=u1 == -1
  If Action Neutral : Subsystem  TreatAsAtomicUnit=on
  If Action Normal : Subsystem  TreatAsAtomicUnit=on
  If Action Reverse : Subsystem  TreatAsAtomicUnit=on
  Merge : Merge  Inputs=3
  OutputTorque = 0 : Constant  Value=0
  Product : Product  InputSameDT=on  SaturateOnIntegerOverflow=on  OutDataTypeStr=Inherit: Same as first input
  Product1 : Product  InputSameDT=on  SaturateOnIntegerOverflow=on  OutDataTypeStr=Inherit: Same as first input
  Transmission Gear ratios : Lookup  InputValues=p.tr_in  Table=p.tr_out  SaturateOnIntegerOverflow=on
  tTransmissionOut_[Nm] : Outport  InitialOutput=0
  nTransmissionIn_[rpm] : Outport  Port=2  InitialOutput=0
  wires:
  GearNr_[-]/1 -> Transmission Gear ratios/1, If/1
  If/3 -> If Action Normal/Action
  If/2 -> If Action Reverse/Action
  If Action Normal/1(Out1) -> Merge/3
  If Action Reverse/1(Out1) -> Merge/2
  If/1 -> If Action Neutral/Action
  If Action Neutral/1(Out1) -> Merge/1
  Product1/1 -> Ensure positive TransmissionRPM/1
  Merge/1 -> tTransmissionOut_[Nm]/1
  Product/1 -> If Action Reverse/1(In1), If Action Normal/1(In1)
  OutputTorque = 0/1 -> If Action Neutral/1(In1)
  Transmission Gear ratios/1 -> Product/2, Product1/1
  nTransmissionOut_[rpm]/1 -> Product1/2
  tTransmissionIn_[Nm]/1 -> Product/1
  Ensure positive TransmissionRPM/1 -> nTransmissionIn_[rpm]/1

== system EMplanner_cs2018a/Audi_A8_Sedan_2/PathFollower_Preview_1/LateralController/CTRL REFERENCES ==
  note: REFERENCE POSITION BASED POSITION CTRL
  Pos x,y,Y [m,m,rad] : Inport
  Position Preview Distance [m] : Inport  Port=2
  TrajOffset [m,m,rad] : Inport  Port=3
  ActorOffset_Left(+) / Right(-)_[m] : Inport  Port=4
  Calculate Lateral Error : Subsystem
      mask Display:
      | port_label('input',1,'pvp');
      | port_label('input',2,'TrajOffset_x_y_Y');
      | port_label('input',3,'ActorOffset_Left_Right');
      | port_label('input',4,'p0');
      | port_label('input',5,'PreviewDistance');
      | port_label('output',1,'dist_psvehicle');
  Calculate Preview Point (pvp) by extrapolating current Vehicle Position (p0) with Preview Distance and Vehicle Orientation : Subsystem
  Find Reference Point (pref0) on Trajectory closest to P0 Point (p0) : Subsystem
      mask Display:
      | port_label('input',1,'pvp');
      | port_label('input',2,'TrajOffset_x_y_Y');
      | port_label('input',3,'ActorOffset_Left_Right');
      | port_label('input',4,'p0');
      | port_label('output',1,'Actor_traj_distance');
      | port_label('output',2,'Actor_traj_angle');
  Mux1 : Mux  Inputs=2
  Selector2 : Selector  InputPortWidth=3  IndexOptions=Index vector (dialog)  Indices=[1 2]  OutputSizes=1
  Terminator : Terminator
  Actor/Traj_distance [m] : Outport
  Actor/Traj_angle [deg] : Outport  Port=2
  e_Lat [m] : Outport  Port=3
  wires:
  Mux1/1 -> Calculate Lateral Error/1(In1), Find Reference Point (pref0) on Trajectory closest to P0 Point (p0)/1(In1)
  Pos x,y,Y [m,m,rad]/1 -> Calculate Preview Point (pvp) by extrapolating current Vehicle Position (p0) with Preview Distance and Vehicle Orientation/2(x,y,Y Demux [m,m,rad]), Find Reference Point (pref0) on Trajectory closest to P0 Point (p0)/4(In4), Selector2/1
  Calculate Preview Point (pvp) by extrapolating current Vehicle Position (p0) with Preview Distance and Vehicle Orientation/1(x_glob_PVP) -> Mux1/1
  Position Preview Distance [m]/1 -> Calculate Lateral Error/5(In5), Calculate Preview Point (pvp) by extrapolating current Vehicle Position (p0) with Preview Distance and Vehicle Orientation/1(Preview Distance)
  Calculate Preview Point (pvp) by extrapolating current Vehicle Position (p0) with Preview Distance and Vehicle Orientation/2(y_glob_PVP) -> Mux1/2
  TrajOffset [m,m,rad]/1 -> Find Reference Point (pref0) on Trajectory closest to P0 Point (p0)/2(In2), Calculate Lateral Error/2(In2)  "L6"
  ActorOffset_Left(+) / Right(-)_[m]/1 -> Find Reference Point (pref0) on Trajectory closest to P0 Point (p0)/3(In3), Calculate Lateral Error/3(In3)
  Find Reference Point (pref0) on Trajectory closest to P0 Point (p0)/1(Out1) -> Actor/Traj_distance [m]/1
  Find Reference Point (pref0) on Trajectory closest to P0 Point (p0)/2(Out2) -> Actor/Traj_angle [deg]/1
  Calculate Preview Point (pvp) by extrapolating current Vehicle Position (p0) with Preview Distance and Vehicle Orientation/3(Y [rad]) -> Terminator/1
  Calculate Lateral Error/1(Out1) -> e_Lat [m]/1
  Selector2/1 -> Calculate Lateral Error/4(In4)

== system EMplanner_cs2018a/Audi_A8_Sedan_2/PathFollower_Preview_1/LateralController/Calculate delta steering error ==
  In1 : Inport
  In2 : Inport  Port=2
  In3 : Inport  Port=3
  In4 : Inport  Port=4
  In5 : Inport  Port=5
  In6 : Inport  Port=6
  In7 : Inport  Port=7
  In8 : Inport  Port=8
  In9 : Inport  Port=9
  In10 : Inport  Port=10
  In11 : Inport  Port=11
  In12 : Inport  Port=12
  eml_delta_steering_error : MATLAB Function  TreatAsAtomicUnit=on  RTWFcnName=sfun_delta_steering_error  RTWFileName=sfun_delta_steering_error
      settings: RTWFileNameOpts=User specified
  Out1 : Outport
  wires:
  In3/1 -> eml_delta_steering_error/3(t_Preview_LatCtrl)
  In2/1 -> eml_delta_steering_error/2(v_x_vehicle_Min)
  In12/1 -> eml_delta_steering_error/12(wheelbase)
  In11/1 -> eml_delta_steering_error/11(Pos_x_CoG_Vehicle)
  In10/1 -> eml_delta_steering_error/10(e_Lat)
  In9/1 -> eml_delta_steering_error/9(inertia_z_vehicle_total)
  In8/1 -> eml_delta_steering_error/8(m_vehicle_total)
  eml_delta_steering_error/1(delta_steeringwheeltotal) -> Out1/1
  In7/1 -> eml_delta_steering_error/7(CorneringStiffness_Tyres_Rear)
  In6/1 -> eml_delta_steering_error/6(CorneringStiffness_Tyres_Front)
  In5/1 -> eml_delta_steering_error/5(yawrate_vehicle)
  In4/1 -> eml_delta_steering_error/4(v_y_vehicle)
  In1/1 -> eml_delta_steering_error/1(v_x_vehicle)

== system EMplanner_cs2018a/Audi_A8_Sedan_2/PathFollower_Preview_1/LateralController/SteeringWheelAngle ==
  Angle_Steering[rad] : Inport
  i_Steering[] : Inport  Port=2
  Angle_SteeringWheel_Last[deg] : Inport  Port=3
  LatCtrl1_Enable[0Off|1On] : Inport  Port=4
  Angle_Max_SteeringWheel[deg]1 : Constant  Value=Angle_Max_SteeringWheel  SampleTime=CSSampleTime
  Const_t_PT1_LatCtrl[s] : Constant  Value=DelayTime  SampleTime=CSSampleTime
  FirstOrderDynamics : Subsystem  mask(First Order Dynamics){}
      mask Display:
      | port_label('input',1,'In')
      | port_label('input',2,'T')
      | port_label('input',3,'Reset')
      | port_label('input',4,'x0')
      | 
      | plot([0.4 0.95], [0.1 0.1]);
      | plot([0.4 0.4], [0.1 0.95]);
      | plot(0.4 + 0.5*[0:0.1:1],0.8- 0.7 * exp(-5*[0:0.1:1]));
  Gain : Gain  SaturateOnIntegerOverflow=on  OutDataTypeStr=Inherit: Same as input  ParamDataTypeStr=Inherit: Same as input
  Product : Product  SaturateOnIntegerOverflow=on  OutDataTypeStr=Inherit: Same as first input
  Rate Limiter : RateLimiter  RisingSlewLimit=MaxSteeringRate  FallingSlewLimit=-MaxSteeringRate  SampleTimeMode=inherited
  Sat_Total : Subsystem
      mask Display:
      | plot([0.25 0.4 0.6 0.75],[0.2 0.2 0.8 0.8])
      | port_label('input',2,'Lim')
      | port_label('output',2,'Info')
  Terminator1 : Terminator
  rad2deg : Gain  Gain=180/pi  SaturateOnIntegerOverflow=on  OutDataTypeStr=Inherit: Same as input  ParamDataTypeStr=Inherit: Same as input
  Angle_SteeringWheel[deg] : Outport
  wires:
  Rate Limiter/1 -> FirstOrderDynamics/1(In)
  Gain/1 -> FirstOrderDynamics/3(Reset)
  Angle_SteeringWheel_Last[deg]/1 -> FirstOrderDynamics/4(x0)
  LatCtrl1_Enable[0Off|1On]/1 -> Gain/1
  Const_t_PT1_LatCtrl[s]/1 -> FirstOrderDynamics/2(TimeConstant[s])
  Sat_Total/2(Sat_Info) -> Terminator1/1
  Angle_Steering[rad]/1 -> rad2deg/1
  i_Steering[]/1 -> Product/2
  rad2deg/1 -> Product/1
  Product/1 -> Sat_Total/1(In)
  Sat_Total/1(Sat_Total) -> Rate Limiter/1
  FirstOrderDynamics/1(Out) -> Angle_SteeringWheel[deg]/1
  Angle_Max_SteeringWheel[deg]1/1 -> Sat_Total/2(Sat_Limit)

== system EMplanner_cs2018a/Audi_A8_Sedan_2/PathFollower_Preview_1/LateralController/s_Preview_LatCtrl ==
  v_x_Vehicle[m|s] : Inport
  v_x_Vehicle_Min[m|s] : Inport  Port=2
  t_Preview_LatCtrl[s] : Inport  Port=3
  Const_s_Preview_LatCtrl_Spacing[0_1] : Constant  Value=[0.1, 0.2, 0.3, 0.4, 0.5, 0.6, 0.7, 0.8,0.9, 1.0]  SampleTime=CSSampleTime
  Max : MinMax  Function=max  Inputs=2  InputSameDT=on  SaturateOnIntegerOverflow=on
  Prod_s_Min : Product  SaturateOnIntegerOverflow=on  OutDataTypeStr=Inherit: Same as first input
  Product : Product  SaturateOnIntegerOverflow=on  OutDataTypeStr=Inherit: Same as first input
  Product1 : Product  SaturateOnIntegerOverflow=on  OutDataTypeStr=Inherit: Same as first input
  s_Preview_LatCtrl[m] : Outport
  wires:
  Prod_s_Min/1 -> Max/2
  v_x_Vehicle_Min[m|s]/1 -> Prod_s_Min/2
  t_Preview_LatCtrl[s]/1 -> Prod_s_Min/1, Product/2
  Const_s_Preview_LatCtrl_Spacing[0_1]/1 -> Product1/2
  Max/1 -> Product1/1
  Product/1 -> Max/1
  v_x_Vehicle[m|s]/1 -> Product/1
  Product1/1 -> s_Preview_LatCtrl[m]/1

== system EMplanner_cs2018a/Audi_A8_Sedan_2/PathFollower_Preview_1/LongitudinalController/Check_Initial_Velocity ==
  " v_actual_[m|s]" : Inport
  Initial_Velocity_[m|s] : Inport  Port=2
  > eps : simulink/Logic and Bit Operations/Compare To Constant  relop=>  const=0.1  OutDataTypeStr=boolean
  Abs : Abs
  Assertion : Assertion  AssertionFailFcn=warningInitialVelocity(blockPath);  StopWhenAssertionFail=off
  Constant : Constant  Value=false
  First ? : Memory  InitialCondition=1
  Logical Operator : Logic  AllPortsSameDT=off  OutDataTypeStr=boolean
  Logical Operator1 : Logic  Operator=NOT  AllPortsSameDT=off  OutDataTypeStr=boolean
  Sum : Sum  Inputs=+-
  wires:
  Logical Operator1/1 -> Assertion/1
  Logical Operator/1 -> Logical Operator1/1
  Constant/1 -> First ?/1
  First ?/1 -> Logical Operator/2
  > eps/1 -> Logical Operator/1
  Sum/1 -> Abs/1
  Abs/1 -> > eps/1
  Initial_Velocity_[m|s]/1 -> Sum/2
  " v_actual_[m|s]"/1 -> Sum/1

== system EMplanner_cs2018a/Audi_A8_Sedan_2/PathFollower_Preview_1/LongitudinalController/If Desired Velocity = 0 ==
  In1 : Inport
  Action Port : ActionPort  InitializeStates=reset  PropagateVarSize=During execution
  constant : Constant  Value=0
  constant1 : Constant  Value=150
  throttle [%] : Outport  InitialOutput=[0]
  brake pressure [bar] : Outport  Port=2  InitialOutput=[150]
  Auto_GearShift : Outport  Port=3
  wires:
  In1/1 -> Auto_GearShift/1
  constant/1 -> throttle [%]/1
  constant1/1 -> brake pressure [bar]/1

== system EMplanner_cs2018a/Audi_A8_Sedan_2/PathFollower_Preview_1/LongitudinalController/If Desired Velocity ~= 0 ==
  note: No brake/throttle actions
      | in case of small ctrl error,
      |  in order to prevent nervous
      | ctrl behaviour
  note: CONSTANT VELOCITY CONTROL
  In1 : Inport
  Desired Velocity [m/s] : Inport  Port=2
  Action Port : ActionPort  InitializeStates=reset  PropagateVarSize=During execution
  Dead Zone1 : DeadZone  LowerValue=-10  UpperValue=1  SaturateOnIntegerOverflow=on
  Gain1 : Gain  Gain=-1
  Gain2 : Gain  Gain=1.5
  Limiter_brake : Saturate  UpperLimit=150  LowerLimit=0
  Limiter_throttle : Saturate  UpperLimit=100  LowerLimit=0
  PID_AWU : Subsystem  mask(PID Controller){P=LongCtrl_P, I=LongCtrl_I, D=LongCtrl_D}
      mask prompts: P "Proportional:"; I "Integral:"; D "Derivative:"
      mask help:
      | Enter expressions for proportional, integral, and derivative terms.
      | P+I/s+Ds
      mask Help: This block implements a PID controller where parameters are entered for the Proportional, Integral and Derivative terms. Unmask this block to see how it works. The derivative term is implemented using a true derivative block.
      mask Display: disp('PID')
  throttle [%] : Outport
  brake pressure [bar] : Outport  Port=2
  Auto_GearShift : Outport  Port=3
  wires:
  Dead Zone1/1 -> Gain2/1, Limiter_throttle/1
  Gain1/1 -> Limiter_brake/1
  Gain2/1 -> Gain1/1
  PID_AWU/1(u) -> Dead Zone1/1
  Desired Velocity [m/s]/1 -> PID_AWU/1(e)
  In1/1 -> Auto_GearShift/1
  Limiter_brake/1 -> brake pressure [bar]/1
  Limiter_throttle/1 -> throttle [%]/1  "throttle"

== system EMplanner_cs2018a/Audi_A8_Sedan_2/PathFollower_Preview_1/LongitudinalController/Memory External IC ==
  note: Xnew
  note: Initial Value
  u : Inport
  IC : Inport  Port=2
  FixPt Constant : Constant  DisableCoverage=on  Value=0  OutDataTypeStr=fixdt(0,8,0)
  FixPt Data Type Duplicate1 : DataTypeDuplicate  DisableCoverage=on  NumInputPorts=3
  Init : Switch  Criteria=u2 ~= 0  OutDataTypeStr=Inherit: Inherit via back propagation  ZeroCross=off
  Memory : Memory  InitialCondition=1  InheritSampleTime=on
  Memory1 : Memory  InheritSampleTime=on
  y : Outport
  wires:
  Memory1/1 -> Init/3  "Xold"
  Init/1 -> y/1, FixPt Data Type Duplicate1/1
  Memory/1 -> Init/2
  FixPt Constant/1 -> Memory/1
  u/1 -> Memory1/1, FixPt Data Type Duplicate1/2
  IC/1 -> Init/1, FixPt Data Type Duplicate1/3

== system EMplanner_cs2018a/Audi_A8_Sedan_2/SELF_Demux/compas converter/cart2compas ==
  Angle [deg] : Inport
  Constant : Constant  Value=90
  Constant1 : Constant  Value=360
  Gain : Gain  Gain=1/360
  Gain1 : Gain  Gain=360
  Gain2 : Gain  Gain=-1
  Rounding Function : Rounding
  Sum : Sum  Inputs=|-+
  Sum1 : Sum  Inputs=-+|
  Sum2 : Sum  Inputs=++|
  heading [deg] : Outport
  wires:
  Gain/1 -> Rounding Function/1
  Rounding Function/1 -> Gain1/1
  Gain1/1 -> Sum/1
  Angle [deg]/1 -> Sum1/2
  Sum/1 -> Gain2/1
  Sum1/1 -> Gain/1, Sum/2
  Constant/1 -> Sum1/1
  Gain2/1 -> Sum2/2
  Constant1/1 -> Sum2/1
  Sum2/1 -> heading [deg]/1

== system EMplanner_cs2018a/Audi_A8_Sedan_1/control module/control main/longitudinal control double PID/discrete pid ==
  err : Inport
  kp : Inport  Port=2
  ki : Inport  Port=3
  kd : Inport  Port=4
  Add2 : Sum  Inputs=+++
  Add3 : Sum
  Add4 : Sum  Inputs=+-
  Delay3 : Delay  DelayLength=1
  Delay4 : Delay  DelayLength=1
  Divide : Product  Inputs=**
  Divide1 : Product  Inputs=**
  Divide2 : Product  Inputs=**
  Gain : Gain  Gain=0.01
  pid_out : Outport
  wires:
  [KD_PID_distance] -> Divide2/2
  err/1 -> Delay4/1, Divide/2, Add3/1, Add4/1
  Divide/1 -> Add2/1
  Divide2/1 -> Add2/3
  Add3/1 -> Gain/1, Divide1/1
  Delay4/1 -> Add4/2
  [KP_PID_distance] -> Divide/1
  Divide1/1 -> Add2/2
  Delay3/1 -> Add3/2
  [KI_PID_distance] -> Divide1/2
  Add4/1 -> Divide2/1
  Add2/1 -> pid_out/1
  kp/1 -> [KP_PID_distance]
  ki/1 -> [KI_PID_distance]
  kd/1 -> [KD_PID_distance]
  Gain/1 -> Delay3/1

== system EMplanner_cs2018a/Audi_A8_Sedan_1/control module/control main/longitudinal control double PID/discrete pid1 ==
  err : Inport
  kp : Inport  Port=2
  ki : Inport  Port=3
  kd : Inport  Port=4
  Add2 : Sum  Inputs=+++
  Add3 : Sum
  Add4 : Sum  Inputs=+-
  Delay3 : Delay  DelayLength=1
  Delay4 : Delay  DelayLength=1
  Divide : Product  Inputs=**
  Divide1 : Product  Inputs=**
  Divide2 : Product  Inputs=**
  Gain : Gain  Gain=0.01
  pid_out : Outport
  wires:
  Gain/1 -> Delay3/1
  kd/1 -> [KD_PID_distance]
  ki/1 -> [KI_PID_distance]
  kp/1 -> [KP_PID_distance]
  Add2/1 -> pid_out/1
  Add4/1 -> Divide2/1
  [KI_PID_distance] -> Divide1/2
  Delay3/1 -> Add3/2
  Divide1/1 -> Add2/2
  [KP_PID_distance] -> Divide/1
  Delay4/1 -> Add4/2
  Add3/1 -> Divide1/1, Gain/1
  Divide2/1 -> Add2/3
  Divide/1 -> Add2/1
  err/1 -> Add4/1, Add3/1, Divide/2, Delay4/1
  [KD_PID_distance] -> Divide2/2

== system EMplanner_cs2018a/Audi_A8_Sedan_2/Dynamics_Simple/Chassis/Bicycle_model_[XYZ]/Fyi --> Fy // Mz ==
  DeltaWheel_[rad] : Inport
  Fy_f_[N] : Inport  Port=2
  Fy_r_[N] : Inport  Port=3
  Fy : Fcn  Expr=u(2)*cos(u(1)) + u(3)
  Mux1 : Mux  Inputs=3
  Mz : Fcn  Expr=u(2)*p.a*cos(u(1)) - u(3)*p.b
  Fy_[N] : Outport  InitialOutput=0
  Mz_[Nm] : Outport  Port=2  InitialOutput=0
  wires:
  DeltaWheel_[rad]/1 -> Mux1/1  "DeltaWheel_[rad]"
  Mz/1 -> Mz_[Nm]/1
  Fy/1 -> Fy_[N]/1
  Mux1/1 -> Mz/1, Fy/1
  Fy_f_[N]/1 -> Mux1/2
  Fy_r_[N]/1 -> Mux1/3
